simulink model "SP_nonlinear_LQR"  (R2016b)
settings: Solver=ode4  StartTime=0.0  StopTime=100  FixedStep=0.001  RelTol=1e-3
values from neighbouring files (symbols this model uses):
  K = lqr(P_sp,Q,R)    [SP_LQG_controller_design.m]
  Ke_sp = K_bar(:,1)    [SP_LQG_controller_design.m]    (also in controller_parameter.mat = -14.1421356237)
  Kx_sp = K_bar(:,2:end)    [SP_LQG_controller_design.m]    (also in controller_parameter.mat = [-9.4028503548 -29.2130812278])
undefined symbols (not defined in the file or in its folder): An, Aqw, Asp1, Bn, Bqw, Bsp1, Cn, Cqw, Csp1, Kn, lin_sys, Nu, Nu_inv, Nx, Ny, op
libraries: aerolibatmos2 x10, aerolib3dof2 x1, aerolib6dof2 x1, aerolibasang x1
(part 2 of 7)

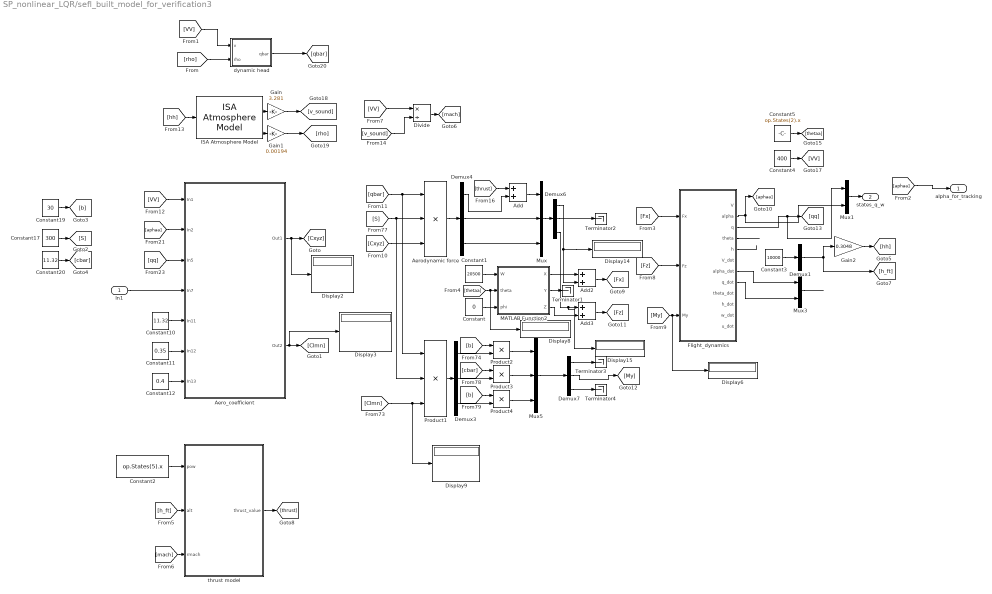
== system SP_nonlinear_LQR/sefl_built_model_for_verification3 ==
  In1 : Inport
  Add : Sum
  Add2 : Sum
  Add3 : Sum
  Aero_coefficient : Subsystem
      mask Display:
      | port_label('input', 1, 'vt')
      | port_label('input', 2, 'alpha')
      | 
      | port_label('input', 3, 'q')
      | 
      | port_label('input', 4, 'el')
      | 
      | 
      | 
      | port_label('input', 5, 'cbar')
      | port_label('input', 6, 'xcgr')
      | port_label('input', 7, 'xcg')
      | port_label('output', 1, 'Cxz')
      | port_label('output', 2, 'Cm')
  "Aerodynamic force " : Product  Inputs=3
  Constant : Constant  Value=0
  Constant1 : Constant  Value=20500
  Constant10 : Constant  Value=11.32
  Constant11 : Constant  Value=0.35
  Constant12 : Constant  Value=0.4
  Constant17 : Constant  Value=300
  Constant19 : Constant  Value=30
  Constant2 : Constant  Value=op.States(5).x
  Constant20 : Constant  Value=11.32
  Constant3 : Constant  Value=10000
  Constant4 : Constant  Value=400
  Constant5 : Constant  Value=op.States(2).x
  Demux1 : Demux  Outputs=1
  Demux{3..4,6..7} (4 alike) : Demux  Outputs=3
  Display{2..3,6,8..9,14..15} (7 alike) : Display
  Divide : Product  Inputs=*/
  Flight_dynamics : Subsystem
  Gain : Gain  Gain=3.281
  Gain1 : Gain  Gain=0.00194
  Gain2 : Gain  Gain=0.3048
  ISA Atmosphere Model : aerolibatmos2/ISA Atmosphere Model  custom=off  g=9.80665  gamma=1.4  R=287.0531  L=0.0065  h_trop=11000  h_strat=20000  rho0=1.225  P0=101325  T0=288.15  h0=0
  MATLAB Function2 : MATLAB Function  TreatAsAtomicUnit=on
  Mux : Mux  Inputs=3
  Mux1 : Mux  Inputs=2
  Mux3 : Mux  Inputs=2
  Mux5 : Mux  Inputs=3
  Product1 : Product  Inputs=3
  Product2 : Product
  Product3 : Product
  Product4 : Product
  Terminator{1..4} (4 alike) : Terminator
  dynamic head : MATLAB Function  TreatAsAtomicUnit=on
  thrust model : MATLAB Function  TreatAsAtomicUnit=on
  alpha_for_tracking : Outport
  states_q_w : Outport  Port=2
  wires:
  [aphaa] -> alpha_for_tracking/1
  Constant5/1 -> [thetaa]
  Constant4/1 -> [VV]
  Constant3/1 -> Demux1/1
  Constant2/1 -> thrust model/1(pow)
  Flight_dynamics/8(q_dot) -> Mux3/2
  Flight_dynamics/7(alpha_dot) -> Mux3/1
  [qq] -> Aero_coefficient/3(In5)
  [aphaa] -> Aero_coefficient/2(In2)
  [VV] -> Aero_coefficient/1(In1)
  Flight_dynamics/5(h) -> ?
  ISA Atmosphere Model/4 -> Gain1/1
  ISA Atmosphere Model/2 -> Gain/1
  [qbar] -> Product1/1, "Aerodynamic force "/1
  In1/1 -> Aero_coefficient/4(In7)
  Product4/1 -> Mux5/3
  Constant10/1 -> Aero_coefficient/5(In11)
  Constant11/1 -> Aero_coefficient/6(In12)
  Mux5/1 -> Demux7/1
  Constant17/1 -> [S]
  Gain1/1 -> [rho]
  Product3/1 -> Mux5/2
  Product2/1 -> Mux5/1
  [VV] -> Divide/1
  [VV] -> dynamic head/1(v)
  Aero_coefficient/1(Out1) -> Display2/1, [Cxyz]
  [rho] -> dynamic head/2(rho)
  Aero_coefficient/2(Out2) -> [Clmn], Display3/1
  Constant20/1 -> [cbar]
  Constant19/1 -> [b]
  Demux1/1 -> Gain2/1, [h_ft]
  [hh] -> ISA Atmosphere Model/1
  Demux4/3 -> Mux/3
  Gain/1 -> [v_sound]
  Divide/1 -> [mach]
  Add/1 -> Mux/1
  Demux4/2 -> Mux/2
  [v_sound] -> Divide/2
  Demux4/1 -> Add/2
  Mux/1 -> Demux6/1
  Constant12/1 -> Aero_coefficient/7(In13)
  Gain2/1 -> [hh]
  dynamic head/1(qbar) -> [qbar]
  thrust model/1(thrust_value) -> [thrust]
  [h_ft] -> thrust model/2(alt)
  [mach] -> thrust model/3(rmach)
  [thrust] -> Add/1
  Demux3/3 -> Product4/2
  [b] -> Product4/1
  "Aerodynamic force "/1 -> Demux4/1
  [Cxyz] -> "Aerodynamic force "/3
  [S] -> "Aerodynamic force "/2, Product1/2
  [Clmn] -> Display9/1, Product1/3
  [b] -> Product2/1
  Product1/1 -> Demux3/1
  Demux3/1 -> Product2/2
  Demux3/2 -> Product3/2
  [cbar] -> Product3/1
  Demux6/3 -> Display15/1, Add3/1
  Demux6/2 -> Terminator2/1
  Demux7/1 -> Terminator3/1
  Demux7/3 -> Terminator4/1
  Constant1/1 -> MATLAB Function2/1(W)
  [thetaa] -> Display8/1, MATLAB Function2/2(theta)
  Constant/1 -> MATLAB Function2/3(phi)
  MATLAB Function2/1(X) -> Add2/1
  Demux6/1 -> Display14/1, Add2/2
  MATLAB Function2/3(Z) -> Add3/2
  MATLAB Function2/2(Y) -> Terminator1/1
  Add2/1 -> [Fx]
  Add3/1 -> [Fz]
  Demux7/2 -> [My]
  [Fx] -> Flight_dynamics/1(Fx)
  [Fz] -> Flight_dynamics/2(Fz)
  [My] -> Flight_dynamics/3(My), Display6/1
  Mux3/1 -> ?
  Flight_dynamics/2(alpha) -> Mux1/2, [aphaa]
  Flight_dynamics/3(q) -> Mux1/1, [qq]
  Flight_dynamics/4(theta) -> ?
  Mux1/1 -> states_q_w/1

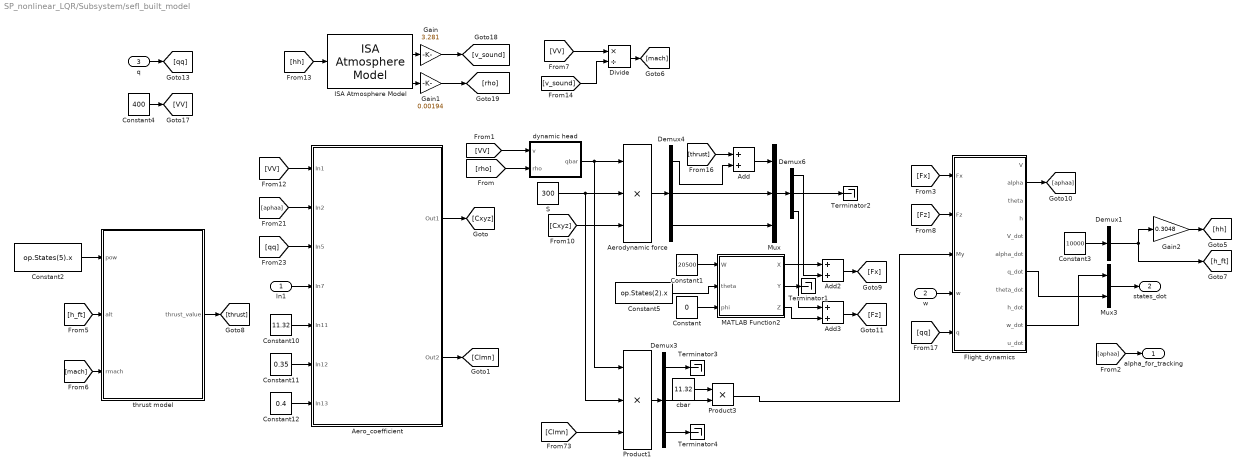
== system SP_nonlinear_LQR/Subsystem/sefl_built_model ==
  In1 : Inport
  w : Inport  Port=2
  q : Inport  Port=3
  Add : Sum
  Add2 : Sum
  Add3 : Sum
  Aero_coefficient : Subsystem
      mask Display:
      | port_label('input', 1, 'vt')
      | port_label('input', 2, 'alpha')
      | 
      | port_label('input', 3, 'q')
      | 
      | port_label('input', 4, 'el')
      | 
      | 
      | 
      | port_label('input', 5, 'cbar')
      | port_label('input', 6, 'xcgr')
      | port_label('input', 7, 'xcg')
      | port_label('output', 1, 'Cxz')
      | port_label('output', 2, 'Cm')
  "Aerodynamic force " : Product  Inputs=3
  Constant : Constant  Value=0
  Constant1 : Constant  Value=20500
  Constant10 : Constant  Value=11.32
  Constant11 : Constant  Value=0.35
  Constant12 : Constant  Value=0.4
  Constant2 : Constant  Value=op.States(5).x
  Constant3 : Constant  Value=10000
  Constant4 : Constant  Value=400
  Constant5 : Constant  Value=op.States(2).x
  Demux1 : Demux  Outputs=1
  Demux3 : Demux  Outputs=3
  Demux4 : Demux  Outputs=3
  Demux6 : Demux  Outputs=3
  Divide : Product  Inputs=*/
  Flight_dynamics : Subsystem
  Gain : Gain  Gain=3.281
  Gain1 : Gain  Gain=0.00194
  Gain2 : Gain  Gain=0.3048
  ISA Atmosphere Model : aerolibatmos2/ISA Atmosphere Model  custom=off  g=9.80665  gamma=1.4  R=287.0531  L=0.0065  h_trop=11000  h_strat=20000  rho0=1.225  P0=101325  T0=288.15  h0=0
  MATLAB Function2 : MATLAB Function  TreatAsAtomicUnit=on
  Mux : Mux  Inputs=3
  Mux3 : Mux  Inputs=2
  Product1 : Product  Inputs=3
  Product3 : Product
  S : Constant  Value=300
  Terminator{1..4} (4 alike) : Terminator
  cbar : Constant  Value=11.32
  dynamic head : MATLAB Function  TreatAsAtomicUnit=on
  thrust model : MATLAB Function  TreatAsAtomicUnit=on
  alpha_for_tracking : Outport
  states_dot : Outport  Port=2
  wires:
  Flight_dynamics/2(alpha) -> [aphaa]
  Mux3/1 -> states_dot/1
  Product3/1 -> Flight_dynamics/3(My)
  [Fz] -> Flight_dynamics/2(Fz)
  [Fx] -> Flight_dynamics/1(Fx)
  Add3/1 -> [Fz]
  Add2/1 -> [Fx]
  MATLAB Function2/2(Y) -> Terminator1/1
  MATLAB Function2/3(Z) -> Add3/2
  Demux6/1 -> Add2/2
  MATLAB Function2/1(X) -> Add2/1
  Constant/1 -> MATLAB Function2/3(phi)
  Constant5/1 -> MATLAB Function2/2(theta)
  Constant1/1 -> MATLAB Function2/1(W)
  Demux6/2 -> Terminator2/1
  Demux6/3 -> Add3/1
  cbar/1 -> Product3/1
  Demux3/2 -> Product3/2
  Product1/1 -> Demux3/1
  [Clmn] -> Product1/3
  S/1 -> Product1/2, "Aerodynamic force "/2
  [Cxyz] -> "Aerodynamic force "/3
  "Aerodynamic force "/1 -> Demux4/1
  [thrust] -> Add/1
  [mach] -> thrust model/3(rmach)
  [h_ft] -> thrust model/2(alt)
  thrust model/1(thrust_value) -> [thrust]
  Gain2/1 -> [hh]
  Constant12/1 -> Aero_coefficient/7(In13)
  Mux/1 -> Demux6/1
  Demux4/1 -> Add/2
  [v_sound] -> Divide/2
  Demux4/2 -> Mux/2
  Add/1 -> Mux/1
  Divide/1 -> [mach]
  Gain/1 -> [v_sound]
  Demux4/3 -> Mux/3
  [hh] -> ISA Atmosphere Model/1
  Demux1/1 -> [h_ft], Gain2/1
  Aero_coefficient/2(Out2) -> [Clmn]
  [rho] -> dynamic head/2(rho)
  Aero_coefficient/1(Out1) -> [Cxyz]
  [VV] -> dynamic head/1(v)
  [VV] -> Divide/1
  Gain1/1 -> [rho]
  Constant11/1 -> Aero_coefficient/6(In12)
  Constant10/1 -> Aero_coefficient/5(In11)
  In1/1 -> Aero_coefficient/4(In7)
  dynamic head/1(qbar) -> "Aerodynamic force "/1, Product1/1
  ISA Atmosphere Model/2 -> Gain/1
  ISA Atmosphere Model/4 -> Gain1/1
  [VV] -> Aero_coefficient/1(In1)
  [aphaa] -> Aero_coefficient/2(In2)
  [qq] -> Aero_coefficient/3(In5)
  q/1 -> [qq]
  Flight_dynamics/10(w_dot) -> Mux3/1
  Flight_dynamics/7(q_dot) -> Mux3/2
  Constant2/1 -> thrust model/1(pow)
  Constant3/1 -> Demux1/1
  Constant4/1 -> [VV]
  [aphaa] -> alpha_for_tracking/1
  w/1 -> Flight_dynamics/4(w)
  [qq] -> Flight_dynamics/5(q)
  Demux3/1 -> Terminator3/1
  Demux3/3 -> Terminator4/1

== system SP_nonlinear_LQR/Subsystem1/Aero_coefficient ==
  In1 : Inport
  In2 : Inport  Port=2
  In5 : Inport  Port=3
  In7 : Inport  Port=4
  In11 : Inport  Port=5
  In12 : Inport  Port=6
  In13 : Inport  Port=7
  Aerodynamic coefficient : MATLAB Function  TreatAsAtomicUnit=on
  Constant : Constant
  Constant1 : Constant
  Constant2 : Constant
  Mux1 : Mux  Inputs=3
  Mux2 : Mux  Inputs=3
  Out1 : Outport
  Out2 : Outport  Port=2
  wires:
  In5/1 -> Aerodynamic coefficient/3(q)
  In1/1 -> Aerodynamic coefficient/1(vt)
  In2/1 -> Aerodynamic coefficient/2(alpha)
  In7/1 -> Aerodynamic coefficient/4(el)
  Aerodynamic coefficient/3(cmt) -> Mux2/2
  In11/1 -> Aerodynamic coefficient/5(cbar)
  In12/1 -> Aerodynamic coefficient/6(xcgr)
  Aerodynamic coefficient/2(czt) -> Mux1/3
  In13/1 -> Aerodynamic coefficient/7(xcg)
  Aerodynamic coefficient/1(cxt) -> Mux1/1
  Mux1/1 -> Out1/1
  Mux2/1 -> Out2/1
  Constant/1 -> Mux1/2
  Constant1/1 -> Mux2/1
  Constant2/1 -> Mux2/3

== system SP_nonlinear_LQR/dynamic_for_linsys1/Aero_coefficient ==
  In1 : Inport
  In2 : Inport  Port=2
  In5 : Inport  Port=3
  In7 : Inport  Port=4
  In11 : Inport  Port=5
  In12 : Inport  Port=6
  In13 : Inport  Port=7
  Aerodynamic coefficient : MATLAB Function  TreatAsAtomicUnit=on
  Constant : Constant
  Constant1 : Constant
  Constant2 : Constant
  Mux1 : Mux  Inputs=3
  Mux2 : Mux  Inputs=3
  Out1 : Outport
  Out2 : Outport  Port=2
  wires:
  In5/1 -> Aerodynamic coefficient/3(q)
  In1/1 -> Aerodynamic coefficient/1(vt)
  In2/1 -> Aerodynamic coefficient/2(alpha)
  In7/1 -> Aerodynamic coefficient/4(el)
  Aerodynamic coefficient/3(cmt) -> Mux2/2
  In11/1 -> Aerodynamic coefficient/5(cbar)
  In12/1 -> Aerodynamic coefficient/6(xcgr)
  Aerodynamic coefficient/2(czt) -> Mux1/3
  In13/1 -> Aerodynamic coefficient/7(xcg)
  Aerodynamic coefficient/1(cxt) -> Mux1/1
  Mux1/1 -> Out1/1
  Mux2/1 -> Out2/1
  Constant/1 -> Mux1/2
  Constant1/1 -> Mux2/1
  Constant2/1 -> Mux2/3

== system SP_nonlinear_LQR/dynamic_for_linsys1/Flight_dynamics ==
  Fx : Inport
  Fz : Inport  Port=2
  My : Inport  Port=3
  Display : Display
  From8 : From  Commented=on  GotoTag=h
  From9 : From  Commented=on  GotoTag=w
  Gain : Gain  Gain=1.57e-3
  Gain1 : Gain  Gain=1.57e-3
  Gain2 : Gain  Gain=1/55814
  Goto15 : Goto  Commented=on  GotoTag=h
  Integrator : Integrator  InitialCondition=op.States(3).x(1)
  Integrator1 : Integrator  InitialCondition=op.States(3).x(2)
  Integrator2 : Integrator
  Integrator3 : Integrator  InitialCondition=op.States(2).x
  Integrator4 : Integrator  Commented=on  InitialCondition=10000
  MATLAB Function : MATLAB Function  TreatAsAtomicUnit=on
  Product : Product
  Product1 : Product
  Sum : Sum  Inputs=|-+
  Sum1 : Sum  Inputs=|++
  V : Outport
  alpha : Outport  Port=2
  q : Outport  Port=3
  theta : Outport  Port=4
  V_dot : Outport  Port=5
  alpha_dot : Outport  Port=6
  q_dot : Outport  Port=7
  theta_dot : Outport  Port=8
  wires:
  Fx/1 -> Gain/1
  Fz/1 -> Gain1/1
  Gain/1 -> [Fx_m]
  Gain1/1 -> [Fz_m]
  My/1 -> Gain2/1
  Gain2/1 -> [My_Iy]
  Product/1 -> Sum/1
  [Fx_m] -> Sum/2
  Sum/1 -> [u_dot], Integrator/1  "u_dot"
  Integrator/1 -> [u], Product1/1  "u"
  Product1/1 -> Sum1/1
  [Fz_m] -> Sum1/2
  Sum1/1 -> [w_dot], Integrator1/1  "w_dot"
  Integrator1/1 -> Integrator4/1, [w]  "w"
  [w] -> Product/2
  [My_Iy] -> [q], Integrator2/1  "q_dot"
  Integrator2/1 -> Product1/2, [q_dot], [theta_dot], Integrator3/1, Product/1  "q"
  Integrator3/1 -> [theta]  "theta"
  [w] -> MATLAB Function/1(w)
  MATLAB Function/2(alpha) -> [alpha]
  [u_dot] -> MATLAB Function/4(u_dot)
  [w_dot] -> MATLAB Function/3(w_dot)
  MATLAB Function/3(alpha_dot) -> [alpha_dot]
  [V] -> Display/1, V/1
  [alpha] -> alpha/1
  [q] -> q/1
  [theta] -> theta/1
  [V_dot] -> V_dot/1
  [alpha_dot] -> alpha_dot/1
  [q_dot] -> q_dot/1
  [theta_dot] -> theta_dot/1
  MATLAB Function/1(V) -> [V]
  MATLAB Function/4(V_dot) -> [V_dot]
  Integrator4/1 -> Goto15/1
  From9/1 -> ?
  [u] -> MATLAB Function/2(u)

== system SP_nonlinear_LQR/q_w_as states/Aero_coefficient ==
  In1 : Inport
  In2 : Inport  Port=2
  In5 : Inport  Port=3
  In7 : Inport  Port=4
  In11 : Inport  Port=5
  In12 : Inport  Port=6
  In13 : Inport  Port=7
  Aerodynamic coefficient : MATLAB Function  TreatAsAtomicUnit=on
  Constant : Constant
  Constant1 : Constant
  Constant2 : Constant
  Mux1 : Mux  Inputs=3
  Mux2 : Mux  Inputs=3
  Out1 : Outport
  Out2 : Outport  Port=2
  wires:
  In5/1 -> Aerodynamic coefficient/3(q)
  In1/1 -> Aerodynamic coefficient/1(vt)
  In2/1 -> Aerodynamic coefficient/2(alpha)
  In7/1 -> Aerodynamic coefficient/4(el)
  Aerodynamic coefficient/3(cmt) -> Mux2/2
  In11/1 -> Aerodynamic coefficient/5(cbar)
  In12/1 -> Aerodynamic coefficient/6(xcgr)
  Aerodynamic coefficient/2(czt) -> Mux1/3
  In13/1 -> Aerodynamic coefficient/7(xcg)
  Aerodynamic coefficient/1(cxt) -> Mux1/1
  Mux1/1 -> Out1/1
  Mux2/1 -> Out2/1
  Constant/1 -> Mux1/2
  Constant1/1 -> Mux2/1
  Constant2/1 -> Mux2/3

== system SP_nonlinear_LQR/q_w_as states/Flight_dynamics ==
  Fx : Inport
  Fz : Inport  Port=2
  My : Inport  Port=3
  Constant : Constant  Value=op.States(3).x(1)
  Constant1 : Constant  Value=0
  Display : Display
  Gain : Gain  Gain=1/637.1604
  Gain1 : Gain  Gain=1/637.1604
  Gain2 : Gain  Gain=1/55814
  Goto15 : Goto  Commented=on  GotoTag=h
  Goto4 : Goto  Commented=on  GotoTag=theta
  Goto5 : Goto  Commented=on  GotoTag=theta_dot
  Integrator1 : Integrator  InitialCondition=op.States(3).x(2)
  Integrator2 : Integrator
  Integrator3 : Integrator  Commented=on  InitialCondition=op.States(2).x
  Integrator4 : Integrator  Commented=on  InitialCondition=10000
  MATLAB Function : MATLAB Function  TreatAsAtomicUnit=on
  Product1 : Product
  Sum1 : Sum  Inputs=|++
  V : Outport
  alpha : Outport  Port=2
  q : Outport  Port=3
  theta : Outport  Port=4
  h : Outport  Port=5
  V_dot : Outport  Port=6
  alpha_dot : Outport  Port=7
  q_dot : Outport  Port=8
  theta_dot : Outport  Port=9
  h_dot : Outport  Port=10
  w_dot : Outport  Port=11
  u_dot : Outport  Port=12
  wires:
  [u] -> Product1/1
  Constant1/1 -> MATLAB Function/4(u_dot)
  Constant/1 -> [u]
  Fx/1 -> Gain/1
  Fz/1 -> Gain1/1
  Gain/1 -> [Fx_m]
  Gain1/1 -> [Fz_m]
  My/1 -> Gain2/1
  Gain2/1 -> [My_Iy]
  Product1/1 -> Sum1/1
  [Fz_m] -> Sum1/2
  Sum1/1 -> Integrator1/1, [w_dot]  "w_dot"
  Integrator1/1 -> Integrator4/1, [w]  "w"
  [My_Iy] -> [q_dot], Integrator2/1  "q_dot"
  Integrator2/1 -> Product1/2, [q], Goto5/1, Integrator3/1  "q"
  Integrator3/1 -> Goto4/1  "theta"
  [w] -> MATLAB Function/1(w)
  MATLAB Function/2(alpha) -> [alpha]
  [w_dot] -> MATLAB Function/3(w_dot)
  MATLAB Function/3(alpha_dot) -> [alpha_dot]
  [V] -> Display/1, V/1
  [alpha] -> alpha/1
  [q] -> q/1
  [theta] -> theta/1
  [V_dot] -> V_dot/1
  [alpha_dot] -> alpha_dot/1
  [q_dot] -> q_dot/1
  [theta_dot] -> theta_dot/1
  MATLAB Function/1(V) -> [V]
  MATLAB Function/4(V_dot) -> [V_dot]
  Integrator4/1 -> Goto15/1
  [h] -> h/1
  [w] -> h_dot/1
  [u] -> MATLAB Function/2(u)
  [w_dot] -> w_dot/1
  [u_dot] -> u_dot/1

== system SP_nonlinear_LQR/q_w_as states1/Aero_coefficient ==
  In1 : Inport
  In2 : Inport  Port=2
  In5 : Inport  Port=3
  In7 : Inport  Port=4
  In11 : Inport  Port=5
  In12 : Inport  Port=6
  In13 : Inport  Port=7
  Aerodynamic coefficient : MATLAB Function  TreatAsAtomicUnit=on
  Constant : Constant
  Constant1 : Constant
  Constant2 : Constant
  Mux1 : Mux  Inputs=3
  Mux2 : Mux  Inputs=3
  Out1 : Outport
  Out2 : Outport  Port=2
  wires:
  In5/1 -> Aerodynamic coefficient/3(q)
  In1/1 -> Aerodynamic coefficient/1(vt)
  In2/1 -> Aerodynamic coefficient/2(alpha)
  In7/1 -> Aerodynamic coefficient/4(el)
  Aerodynamic coefficient/3(cmt) -> Mux2/2
  In11/1 -> Aerodynamic coefficient/5(cbar)
  In12/1 -> Aerodynamic coefficient/6(xcgr)
  Aerodynamic coefficient/2(czt) -> Mux1/3
  In13/1 -> Aerodynamic coefficient/7(xcg)
  Aerodynamic coefficient/1(cxt) -> Mux1/1
  Mux1/1 -> Out1/1
  Mux2/1 -> Out2/1
  Constant/1 -> Mux1/2
  Constant1/1 -> Mux2/1
  Constant2/1 -> Mux2/3

== system SP_nonlinear_LQR/q_w_as states1/Flight_dynamics ==
  Fx : Inport
  Fz : Inport  Port=2
  My : Inport  Port=3
  Constant : Constant  Value=op.States(3).x(1)
  Constant1 : Constant  Value=0
  Display : Display
  Gain : Gain  Gain=1/637.1604
  Gain1 : Gain  Gain=1/637.1604
  Gain2 : Gain  Gain=1/55814
  Goto15 : Goto  Commented=on  GotoTag=h
  Goto4 : Goto  Commented=on  GotoTag=theta
  Goto5 : Goto  Commented=on  GotoTag=theta_dot
  Integrator1 : Integrator  InitialCondition=op.States(3).x(2)
  Integrator2 : Integrator
  Integrator3 : Integrator  Commented=on  InitialCondition=op.States(2).x
  Integrator4 : Integrator  Commented=on  InitialCondition=10000
  MATLAB Function : MATLAB Function  TreatAsAtomicUnit=on
  Product1 : Product
  Sum1 : Sum  Inputs=|++
  V : Outport
  alpha : Outport  Port=2
  q : Outport  Port=3
  theta : Outport  Port=4
  h : Outport  Port=5
  V_dot : Outport  Port=6
  alpha_dot : Outport  Port=7
  q_dot : Outport  Port=8
  theta_dot : Outport  Port=9
  h_dot : Outport  Port=10
  w_dot : Outport  Port=11
  u_dot : Outport  Port=12
  wires:
  [u] -> Product1/1
  Constant1/1 -> MATLAB Function/4(u_dot)
  Constant/1 -> [u]
  Fx/1 -> Gain/1
  Fz/1 -> Gain1/1
  Gain/1 -> [Fx_m]
  Gain1/1 -> [Fz_m]
  My/1 -> Gain2/1
  Gain2/1 -> [My_Iy]
  Product1/1 -> Sum1/1
  [Fz_m] -> Sum1/2
  Sum1/1 -> Integrator1/1, [w_dot]  "w_dot"
  Integrator1/1 -> Integrator4/1, [w]  "w"
  [My_Iy] -> [q_dot], Integrator2/1  "q_dot"
  Integrator2/1 -> Product1/2, [q], Goto5/1, Integrator3/1  "q"
  Integrator3/1 -> Goto4/1  "theta"
  [w] -> MATLAB Function/1(w)
  MATLAB Function/2(alpha) -> [alpha]
  [w_dot] -> MATLAB Function/3(w_dot)
  MATLAB Function/3(alpha_dot) -> [alpha_dot]
  [V] -> Display/1, V/1
  [alpha] -> alpha/1
  [q] -> q/1
  [theta] -> theta/1
  [V_dot] -> V_dot/1
  [alpha_dot] -> alpha_dot/1
  [q_dot] -> q_dot/1
  [theta_dot] -> theta_dot/1
  MATLAB Function/1(V) -> [V]
  MATLAB Function/4(V_dot) -> [V_dot]
  Integrator4/1 -> Goto15/1
  [h] -> h/1
  [w] -> h_dot/1
  [u] -> MATLAB Function/2(u)
  [w_dot] -> w_dot/1
  [u_dot] -> u_dot/1

== system SP_nonlinear_LQR/q_w_as states2/Aero_coefficient ==
  In1 : Inport
  In2 : Inport  Port=2
  In5 : Inport  Port=3
  In7 : Inport  Port=4
  In11 : Inport  Port=5
  In12 : Inport  Port=6
  In13 : Inport  Port=7
  Aerodynamic coefficient : MATLAB Function  TreatAsAtomicUnit=on
  Constant : Constant
  Constant1 : Constant
  Constant2 : Constant
  Mux1 : Mux  Inputs=3
  Mux2 : Mux  Inputs=3
  Out1 : Outport
  Out2 : Outport  Port=2
  wires:
  In5/1 -> Aerodynamic coefficient/3(q)
  In1/1 -> Aerodynamic coefficient/1(vt)
  In2/1 -> Aerodynamic coefficient/2(alpha)
  In7/1 -> Aerodynamic coefficient/4(el)
  Aerodynamic coefficient/3(cmt) -> Mux2/2
  In11/1 -> Aerodynamic coefficient/5(cbar)
  In12/1 -> Aerodynamic coefficient/6(xcgr)
  Aerodynamic coefficient/2(czt) -> Mux1/3
  In13/1 -> Aerodynamic coefficient/7(xcg)
  Aerodynamic coefficient/1(cxt) -> Mux1/1
  Mux1/1 -> Out1/1
  Mux2/1 -> Out2/1
  Constant/1 -> Mux1/2
  Constant1/1 -> Mux2/1
  Constant2/1 -> Mux2/3

== system SP_nonlinear_LQR/q_w_as states2/Flight_dynamics ==
  Fx : Inport
  Fz : Inport  Port=2
  My : Inport  Port=3
  Constant : Constant  Value=op.States(3).x(1)
  Constant1 : Constant  Value=0
  Display : Display
  Gain : Gain  Gain=1/637.1604
  Gain1 : Gain  Gain=1/637.1604
  Gain2 : Gain  Gain=1/55814
  Goto15 : Goto  Commented=on  GotoTag=h
  Goto4 : Goto  Commented=on  GotoTag=theta
  Goto5 : Goto  Commented=on  GotoTag=theta_dot
  Integrator1 : Integrator  InitialCondition=op.States(3).x(2)
  Integrator2 : Integrator
  Integrator3 : Integrator  Commented=on  InitialCondition=op.States(2).x
  Integrator4 : Integrator  Commented=on  InitialCondition=10000
  MATLAB Function : MATLAB Function  TreatAsAtomicUnit=on
  Product1 : Product
  Sum1 : Sum  Inputs=|++
  V : Outport
  alpha : Outport  Port=2
  q : Outport  Port=3
  theta : Outport  Port=4
  h : Outport  Port=5
  V_dot : Outport  Port=6
  alpha_dot : Outport  Port=7
  q_dot : Outport  Port=8
  theta_dot : Outport  Port=9
  h_dot : Outport  Port=10
  w_dot : Outport  Port=11
  u_dot : Outport  Port=12
  wires:
  [u] -> Product1/1
  Constant1/1 -> MATLAB Function/4(u_dot)
  Constant/1 -> [u]
  Fx/1 -> Gain/1
  Fz/1 -> Gain1/1
  Gain/1 -> [Fx_m]
  Gain1/1 -> [Fz_m]
  My/1 -> Gain2/1
  Gain2/1 -> [My_Iy]
  Product1/1 -> Sum1/1
  [Fz_m] -> Sum1/2
  Sum1/1 -> Integrator1/1, [w_dot]  "w_dot"
  Integrator1/1 -> Integrator4/1, [w]  "w"
  [My_Iy] -> [q_dot], Integrator2/1  "q_dot"
  Integrator2/1 -> Product1/2, [q], Goto5/1, Integrator3/1  "q"
  Integrator3/1 -> Goto4/1  "theta"
  [w] -> MATLAB Function/1(w)
  MATLAB Function/2(alpha) -> [alpha]
  [w_dot] -> MATLAB Function/3(w_dot)
  MATLAB Function/3(alpha_dot) -> [alpha_dot]
  [V] -> Display/1, V/1
  [alpha] -> alpha/1
  [q] -> q/1
  [theta] -> theta/1
  [V_dot] -> V_dot/1
  [alpha_dot] -> alpha_dot/1
  [q_dot] -> q_dot/1
  [theta_dot] -> theta_dot/1
  MATLAB Function/1(V) -> [V]
  MATLAB Function/4(V_dot) -> [V_dot]
  Integrator4/1 -> Goto15/1
  [h] -> h/1
  [w] -> h_dot/1
  [u] -> MATLAB Function/2(u)
  [w_dot] -> w_dot/1
  [u_dot] -> u_dot/1

== system SP_nonlinear_LQR/q_w_as states3/Aero_coefficient ==
  In1 : Inport
  In2 : Inport  Port=2
  In5 : Inport  Port=3
  In7 : Inport  Port=4
  In11 : Inport  Port=5
  In12 : Inport  Port=6
  In13 : Inport  Port=7
  Aerodynamic coefficient : MATLAB Function  TreatAsAtomicUnit=on
  Constant : Constant
  Constant1 : Constant
  Constant2 : Constant
  Mux1 : Mux  Inputs=3
  Mux2 : Mux  Inputs=3
  Out1 : Outport
  Out2 : Outport  Port=2
  wires:
  In5/1 -> Aerodynamic coefficient/3(q)
  In1/1 -> Aerodynamic coefficient/1(vt)
  In2/1 -> Aerodynamic coefficient/2(alpha)
  In7/1 -> Aerodynamic coefficient/4(el)
  Aerodynamic coefficient/3(cmt) -> Mux2/2
  In11/1 -> Aerodynamic coefficient/5(cbar)
  In12/1 -> Aerodynamic coefficient/6(xcgr)
  Aerodynamic coefficient/2(czt) -> Mux1/3
  In13/1 -> Aerodynamic coefficient/7(xcg)
  Aerodynamic coefficient/1(cxt) -> Mux1/1
  Mux1/1 -> Out1/1
  Mux2/1 -> Out2/1
  Constant/1 -> Mux1/2
  Constant1/1 -> Mux2/1
  Constant2/1 -> Mux2/3

== system SP_nonlinear_LQR/q_w_as states3/Flight_dynamics ==
  Fx : Inport
  Fz : Inport  Port=2
  My : Inport  Port=3
  Constant : Constant  Value=op.States(3).x(1)
  Constant1 : Constant  Value=0
  Display : Display
  Gain : Gain  Gain=1/637.1604
  Gain1 : Gain  Gain=1/637.1604
  Gain2 : Gain  Gain=1/55814
  Goto15 : Goto  Commented=on  GotoTag=h
  Goto4 : Goto  Commented=on  GotoTag=theta
  Goto5 : Goto  Commented=on  GotoTag=theta_dot
  Integrator1 : Integrator  InitialCondition=op.States(3).x(2)
  Integrator2 : Integrator
  Integrator3 : Integrator  Commented=on  InitialCondition=op.States(2).x
  Integrator4 : Integrator  Commented=on  InitialCondition=10000
  MATLAB Function : MATLAB Function  TreatAsAtomicUnit=on
  Product1 : Product
  Sum1 : Sum  Inputs=|++
  V : Outport
  alpha : Outport  Port=2
  q : Outport  Port=3
  theta : Outport  Port=4
  h : Outport  Port=5
  V_dot : Outport  Port=6
  alpha_dot : Outport  Port=7
  q_dot : Outport  Port=8
  theta_dot : Outport  Port=9
  h_dot : Outport  Port=10
  w_dot : Outport  Port=11
  u_dot : Outport  Port=12
  wires:
  [u] -> Product1/1
  Constant1/1 -> MATLAB Function/4(u_dot)
  Constant/1 -> [u]
  Fx/1 -> Gain/1
  Fz/1 -> Gain1/1
  Gain/1 -> [Fx_m]
  Gain1/1 -> [Fz_m]
  My/1 -> Gain2/1
  Gain2/1 -> [My_Iy]
  Product1/1 -> Sum1/1
  [Fz_m] -> Sum1/2
  Sum1/1 -> Integrator1/1, [w_dot]  "w_dot"
  Integrator1/1 -> Integrator4/1, [w]  "w"
  [My_Iy] -> [q_dot], Integrator2/1  "q_dot"
  Integrator2/1 -> Product1/2, [q], Goto5/1, Integrator3/1  "q"
  Integrator3/1 -> Goto4/1  "theta"
  [w] -> MATLAB Function/1(w)
  MATLAB Function/2(alpha) -> [alpha]
  [w_dot] -> MATLAB Function/3(w_dot)
  MATLAB Function/3(alpha_dot) -> [alpha_dot]
  [V] -> Display/1, V/1
  [alpha] -> alpha/1
  [q] -> q/1
  [theta] -> theta/1
  [V_dot] -> V_dot/1
  [alpha_dot] -> alpha_dot/1
  [q_dot] -> q_dot/1
  [theta_dot] -> theta_dot/1
  MATLAB Function/1(V) -> [V]
  MATLAB Function/4(V_dot) -> [V_dot]
  Integrator4/1 -> Goto15/1
  [h] -> h/1
  [w] -> h_dot/1
  [u] -> MATLAB Function/2(u)
  [w_dot] -> w_dot/1
  [u_dot] -> u_dot/1

== system SP_nonlinear_LQR/sefl_built_model_for_verification1/Aero_coefficient ==
  In1 : Inport
  In2 : Inport  Port=2
  In5 : Inport  Port=3
  In7 : Inport  Port=4
  In11 : Inport  Port=5
  In12 : Inport  Port=6
  In13 : Inport  Port=7
  Aerodynamic coefficient : MATLAB Function  TreatAsAtomicUnit=on
  Constant : Constant
  Constant1 : Constant
  Constant2 : Constant
  Mux1 : Mux  Inputs=3
  Mux2 : Mux  Inputs=3
  Out1 : Outport
  Out2 : Outport  Port=2
  wires:
  Constant2/1 -> Mux2/3
  Constant1/1 -> Mux2/1
  Constant/1 -> Mux1/2
  Mux2/1 -> Out2/1
  Mux1/1 -> Out1/1
  Aerodynamic coefficient/1(cxt) -> Mux1/1
  In13/1 -> Aerodynamic coefficient/7(xcg)
  Aerodynamic coefficient/2(czt) -> Mux1/3
  In12/1 -> Aerodynamic coefficient/6(xcgr)
  In11/1 -> Aerodynamic coefficient/5(cbar)
  Aerodynamic coefficient/3(cmt) -> Mux2/2
  In7/1 -> Aerodynamic coefficient/4(el)
  In2/1 -> Aerodynamic coefficient/2(alpha)
  In1/1 -> Aerodynamic coefficient/1(vt)
  In5/1 -> Aerodynamic coefficient/3(q)

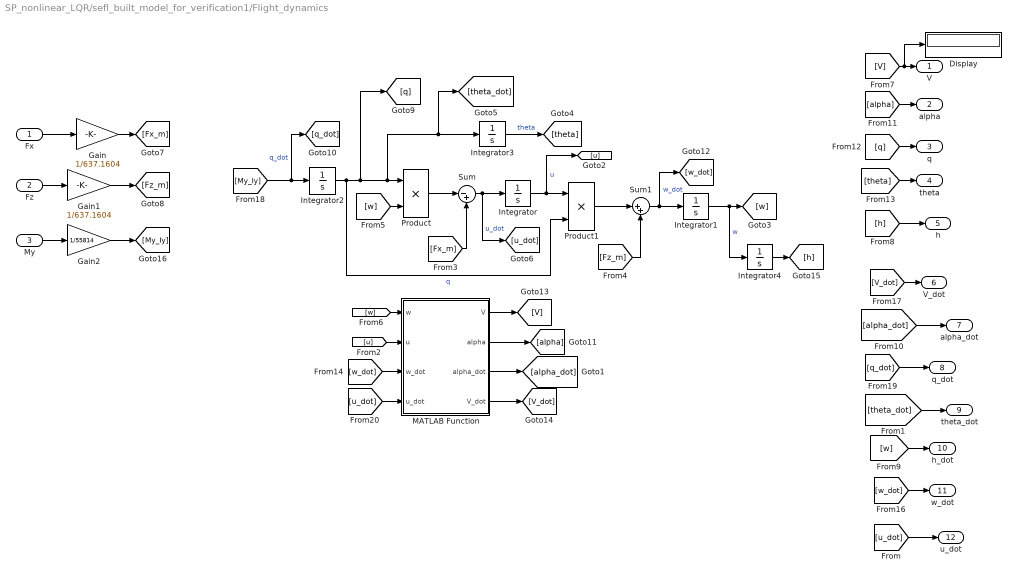
== system SP_nonlinear_LQR/sefl_built_model_for_verification1/Flight_dynamics ==
  Fx : Inport
  Fz : Inport  Port=2
  My : Inport  Port=3
  Display : Display
  Gain : Gain  Gain=1/637.1604
  Gain1 : Gain  Gain=1/637.1604
  Gain2 : Gain  Gain=1/55814
  Integrator : Integrator  InitialCondition=op.States(3).x(1)
  Integrator1 : Integrator  InitialCondition=op.States(3).x(2)
  Integrator2 : Integrator
  Integrator3 : Integrator  InitialCondition=op.States(2).x
  Integrator4 : Integrator  InitialCondition=10000
  MATLAB Function : MATLAB Function  TreatAsAtomicUnit=on
  Product : Product
  Product1 : Product
  Sum : Sum  Inputs=|-+
  Sum1 : Sum  Inputs=|++
  V : Outport
  alpha : Outport  Port=2
  q : Outport  Port=3
  theta : Outport  Port=4
  h : Outport  Port=5
  V_dot : Outport  Port=6
  alpha_dot : Outport  Port=7
  q_dot : Outport  Port=8
  theta_dot : Outport  Port=9
  h_dot : Outport  Port=10
  w_dot : Outport  Port=11
  u_dot : Outport  Port=12
  wires:
  [u_dot] -> u_dot/1
  [w_dot] -> w_dot/1
  [u] -> MATLAB Function/2(u)
  [w] -> h_dot/1
  [h] -> h/1
  Integrator4/1 -> [h]
  MATLAB Function/4(V_dot) -> [V_dot]
  MATLAB Function/1(V) -> [V]
  [theta_dot] -> theta_dot/1
  [q_dot] -> q_dot/1
  [alpha_dot] -> alpha_dot/1
  [V_dot] -> V_dot/1
  [theta] -> theta/1
  [q] -> q/1
  [alpha] -> alpha/1
  [V] -> V/1, Display/1
  MATLAB Function/3(alpha_dot) -> [alpha_dot]
  [w_dot] -> MATLAB Function/3(w_dot)
  [u_dot] -> MATLAB Function/4(u_dot)
  MATLAB Function/2(alpha) -> [alpha]
  [w] -> MATLAB Function/1(w)
  Integrator3/1 -> [theta]  "theta"
  Integrator2/1 -> Product/1, Integrator3/1, [theta_dot], [q], Product1/2  "q"
  [My_Iy] -> Integrator2/1, [q_dot]  "q_dot"
  [w] -> Product/2
  Integrator1/1 -> [w], Integrator4/1  "w"
  Sum1/1 -> Integrator1/1, [w_dot]  "w_dot"
  [Fz_m] -> Sum1/2
  Product1/1 -> Sum1/1
  Integrator/1 -> Product1/1, [u]  "u"
  Sum/1 -> Integrator/1, [u_dot]  "u_dot"
  [Fx_m] -> Sum/2
  Product/1 -> Sum/1
  Gain2/1 -> [My_Iy]
  My/1 -> Gain2/1
  Gain1/1 -> [Fz_m]
  Gain/1 -> [Fx_m]
  Fz/1 -> Gain1/1
  Fx/1 -> Gain/1

== system SP_nonlinear_LQR/sefl_built_model_for_verification2/Aero_coefficient ==
  In1 : Inport
  In2 : Inport  Port=2
  In5 : Inport  Port=3
  In7 : Inport  Port=4
  In11 : Inport  Port=5
  In12 : Inport  Port=6
  In13 : Inport  Port=7
  Aerodynamic coefficient : MATLAB Function  TreatAsAtomicUnit=on
  Constant : Constant
  Constant1 : Constant
  Constant2 : Constant
  Mux1 : Mux  Inputs=3
  Mux2 : Mux  Inputs=3
  Out1 : Outport
  Out2 : Outport  Port=2
  wires:
  In5/1 -> Aerodynamic coefficient/3(q)
  In1/1 -> Aerodynamic coefficient/1(vt)
  In2/1 -> Aerodynamic coefficient/2(alpha)
  In7/1 -> Aerodynamic coefficient/4(el)
  Aerodynamic coefficient/3(cmt) -> Mux2/2
  In11/1 -> Aerodynamic coefficient/5(cbar)
  In12/1 -> Aerodynamic coefficient/6(xcgr)
  Aerodynamic coefficient/2(czt) -> Mux1/3
  In13/1 -> Aerodynamic coefficient/7(xcg)
  Aerodynamic coefficient/1(cxt) -> Mux1/1
  Mux1/1 -> Out1/1
  Mux2/1 -> Out2/1
  Constant/1 -> Mux1/2
  Constant1/1 -> Mux2/1
  Constant2/1 -> Mux2/3

== system SP_nonlinear_LQR/sefl_built_model_for_verification2/Flight_dynamics ==
  Fx : Inport
  Fz : Inport  Port=2
  My : Inport  Port=3
  Constant : Constant  Value=op.States(3).x(1)
  Constant1 : Constant  Value=0
  Display : Display
  Gain : Gain  Gain=1/637.1604
  Gain1 : Gain  Gain=1/637.1604
  Gain2 : Gain  Gain=1/55814
  Goto15 : Goto  Commented=on  GotoTag=h
  Goto4 : Goto  Commented=on  GotoTag=theta
  Goto5 : Goto  Commented=on  GotoTag=theta_dot
  Integrator1 : Integrator  InitialCondition=op.States(3).x(2)
  Integrator2 : Integrator
  Integrator3 : Integrator  Commented=on  InitialCondition=op.States(2).x
  Integrator4 : Integrator  Commented=on  InitialCondition=10000
  MATLAB Function : MATLAB Function  TreatAsAtomicUnit=on
  Product1 : Product
  Sum1 : Sum  Inputs=|++
  V : Outport
  alpha : Outport  Port=2
  q : Outport  Port=3
  theta : Outport  Port=4
  h : Outport  Port=5
  V_dot : Outport  Port=6
  alpha_dot : Outport  Port=7
  q_dot : Outport  Port=8
  theta_dot : Outport  Port=9
  h_dot : Outport  Port=10
  w_dot : Outport  Port=11
  u_dot : Outport  Port=12
  wires:
  [u] -> Product1/1
  Constant1/1 -> MATLAB Function/4(u_dot)
  Constant/1 -> [u]
  Fx/1 -> Gain/1
  Fz/1 -> Gain1/1
  Gain/1 -> [Fx_m]
  Gain1/1 -> [Fz_m]
  My/1 -> Gain2/1
  Gain2/1 -> [My_Iy]
  Product1/1 -> Sum1/1
  [Fz_m] -> Sum1/2
  Sum1/1 -> Integrator1/1, [w_dot]  "w_dot"
  Integrator1/1 -> Integrator4/1, [w]  "w"
  [My_Iy] -> [q_dot], Integrator2/1  "q_dot"
  Integrator2/1 -> Product1/2, [q], Goto5/1, Integrator3/1  "q"
  Integrator3/1 -> Goto4/1  "theta"
  [w] -> MATLAB Function/1(w)
  MATLAB Function/2(alpha) -> [alpha]
  [w_dot] -> MATLAB Function/3(w_dot)
  MATLAB Function/3(alpha_dot) -> [alpha_dot]
  [V] -> Display/1, V/1
  [alpha] -> alpha/1
  [q] -> q/1
  [theta] -> theta/1
  [V_dot] -> V_dot/1
  [alpha_dot] -> alpha_dot/1
  [q_dot] -> q_dot/1
  [theta_dot] -> theta_dot/1
  MATLAB Function/1(V) -> [V]
  MATLAB Function/4(V_dot) -> [V_dot]
  Integrator4/1 -> Goto15/1
  [h] -> h/1
  [w] -> h_dot/1
  [u] -> MATLAB Function/2(u)
  [w_dot] -> w_dot/1
  [u_dot] -> u_dot/1

== system SP_nonlinear_LQR/sefl_built_model_for_verification3/Aero_coefficient ==
  In1 : Inport
  In2 : Inport  Port=2
  In5 : Inport  Port=3
  In7 : Inport  Port=4
  In11 : Inport  Port=5
  In12 : Inport  Port=6
  In13 : Inport  Port=7
  Aerodynamic coefficient : MATLAB Function  TreatAsAtomicUnit=on
  Constant : Constant
  Constant1 : Constant
  Constant2 : Constant
  Mux1 : Mux  Inputs=3
  Mux2 : Mux  Inputs=3
  Out1 : Outport
  Out2 : Outport  Port=2
  wires:
  In5/1 -> Aerodynamic coefficient/3(q)
  In1/1 -> Aerodynamic coefficient/1(vt)
  In2/1 -> Aerodynamic coefficient/2(alpha)
  In7/1 -> Aerodynamic coefficient/4(el)
  Aerodynamic coefficient/3(cmt) -> Mux2/2
  In11/1 -> Aerodynamic coefficient/5(cbar)
  In12/1 -> Aerodynamic coefficient/6(xcgr)
  Aerodynamic coefficient/2(czt) -> Mux1/3
  In13/1 -> Aerodynamic coefficient/7(xcg)
  Aerodynamic coefficient/1(cxt) -> Mux1/1
  Mux1/1 -> Out1/1
  Mux2/1 -> Out2/1
  Constant/1 -> Mux1/2
  Constant1/1 -> Mux2/1
  Constant2/1 -> Mux2/3

== system SP_nonlinear_LQR/sefl_built_model_for_verification3/Flight_dynamics ==
  Fx : Inport
  Fz : Inport  Port=2
  My : Inport  Port=3
  Constant : Constant  Value=op.States(3).x(1)
  Constant1 : Constant  Value=0
  Display : Display
  Gain : Gain  Gain=1/637.1604
  Gain1 : Gain  Gain=1/637.1604
  Gain2 : Gain  Gain=1/55814
  Goto15 : Goto  Commented=on  GotoTag=h
  Goto4 : Goto  Commented=on  GotoTag=theta
  Goto5 : Goto  Commented=on  GotoTag=theta_dot
  Integrator1 : Integrator  InitialCondition=op.States(3).x(2)
  Integrator2 : Integrator
  Integrator3 : Integrator  Commented=on  InitialCondition=op.States(2).x
  Integrator4 : Integrator  Commented=on  InitialCondition=10000
  MATLAB Function : MATLAB Function  TreatAsAtomicUnit=on
  Product1 : Product
  Sum1 : Sum  Inputs=|++
  V : Outport
  alpha : Outport  Port=2
  q : Outport  Port=3
  theta : Outport  Port=4
  h : Outport  Port=5
  V_dot : Outport  Port=6
  alpha_dot : Outport  Port=7
  q_dot : Outport  Port=8
  theta_dot : Outport  Port=9
  h_dot : Outport  Port=10
  w_dot : Outport  Port=11
  u_dot : Outport  Port=12
  wires:
  [u] -> Product1/1
  Constant1/1 -> MATLAB Function/4(u_dot)
  Constant/1 -> [u]
  Fx/1 -> Gain/1
  Fz/1 -> Gain1/1
  Gain/1 -> [Fx_m]
  Gain1/1 -> [Fz_m]
  My/1 -> Gain2/1
  Gain2/1 -> [My_Iy]
  Product1/1 -> Sum1/1
  [Fz_m] -> Sum1/2
  Sum1/1 -> Integrator1/1, [w_dot]  "w_dot"
  Integrator1/1 -> Integrator4/1, [w]  "w"
  [My_Iy] -> [q_dot], Integrator2/1  "q_dot"
  Integrator2/1 -> Product1/2, [q], Goto5/1, Integrator3/1  "q"
  Integrator3/1 -> Goto4/1  "theta"
  [w] -> MATLAB Function/1(w)
  MATLAB Function/2(alpha) -> [alpha]
  [w_dot] -> MATLAB Function/3(w_dot)
  MATLAB Function/3(alpha_dot) -> [alpha_dot]
  [V] -> Display/1, V/1
  [alpha] -> alpha/1
  [q] -> q/1
  [theta] -> theta/1
  [V_dot] -> V_dot/1
  [alpha_dot] -> alpha_dot/1
  [q_dot] -> q_dot/1
  [theta_dot] -> theta_dot/1
  MATLAB Function/1(V) -> [V]
  MATLAB Function/4(V_dot) -> [V_dot]
  Integrator4/1 -> Goto15/1
  [h] -> h/1
  [w] -> h_dot/1
  [u] -> MATLAB Function/2(u)
  [w_dot] -> w_dot/1
  [u_dot] -> u_dot/1

== system SP_nonlinear_LQR/Subsystem/sefl_built_model/Aero_coefficient ==
  In1 : Inport
  In2 : Inport  Port=2
  In5 : Inport  Port=3
  In7 : Inport  Port=4
  In11 : Inport  Port=5
  In12 : Inport  Port=6
  In13 : Inport  Port=7
  Aerodynamic coefficient : MATLAB Function  TreatAsAtomicUnit=on
  Constant : Constant
  Constant1 : Constant
  Constant2 : Constant
  Mux1 : Mux  Inputs=3
  Mux2 : Mux  Inputs=3
  Out1 : Outport
  Out2 : Outport  Port=2
  wires:
  Constant2/1 -> Mux2/3
  Constant1/1 -> Mux2/1
  Constant/1 -> Mux1/2
  Mux2/1 -> Out2/1
  Mux1/1 -> Out1/1
  Aerodynamic coefficient/1(cxt) -> Mux1/1
  In13/1 -> Aerodynamic coefficient/7(xcg)
  Aerodynamic coefficient/2(czt) -> Mux1/3
  In12/1 -> Aerodynamic coefficient/6(xcgr)
  In11/1 -> Aerodynamic coefficient/5(cbar)
  Aerodynamic coefficient/3(cmt) -> Mux2/2
  In7/1 -> Aerodynamic coefficient/4(el)
  In2/1 -> Aerodynamic coefficient/2(alpha)
  In1/1 -> Aerodynamic coefficient/1(vt)
  In5/1 -> Aerodynamic coefficient/3(q)

== system SP_nonlinear_LQR/Subsystem/sefl_built_model/Flight_dynamics ==
  Fx : Inport
  Fz : Inport  Port=2
  My : Inport  Port=3
  w : Inport  Port=4
  q : Inport  Port=5
  Constant : Constant  Value=op.States(3).x(1)
  Constant1 : Constant  Value=0
  Display : Display
  Gain : Gain  Gain=1/637.1604
  Gain1 : Gain  Gain=1/637.1604
  Gain2 : Gain  Gain=1/55814
  MATLAB Function : MATLAB Function  TreatAsAtomicUnit=on
  Product1 : Product
  Sum1 : Sum  Inputs=|++
  V : Outport
  alpha : Outport  Port=2
  theta : Outport  Port=3
  h : Outport  Port=4
  V_dot : Outport  Port=5
  alpha_dot : Outport  Port=6
  q_dot : Outport  Port=7
  theta_dot : Outport  Port=8
  h_dot : Outport  Port=9
  w_dot : Outport  Port=10
  u_dot : Outport  Port=11
  wires:
  [u_dot] -> u_dot/1
  [w_dot] -> w_dot/1
  [u] -> MATLAB Function/2(u)
  [W] -> h_dot/1
  [h] -> h/1
  MATLAB Function/4(V_dot) -> [V_dot]
  MATLAB Function/1(V) -> [V]
  [theta_dot] -> theta_dot/1
  [q_dot] -> q_dot/1
  [alpha_dot] -> alpha_dot/1
  [V_dot] -> V_dot/1
  [theta] -> theta/1
  [alpha] -> alpha/1
  [V] -> V/1, Display/1
  MATLAB Function/3(alpha_dot) -> [alpha_dot]
  [w_dot] -> MATLAB Function/3(w_dot)
  MATLAB Function/2(alpha) -> [alpha]
  [W] -> MATLAB Function/1(w)
  [My_Iy] -> [q_dot]  "q_dot"
  Sum1/1 -> [w_dot]
  [Fz_m] -> Sum1/2
  Product1/1 -> Sum1/1
  Gain2/1 -> [My_Iy]
  My/1 -> Gain2/1
  Gain1/1 -> [Fz_m]
  Gain/1 -> [Fx_m]
  Fz/1 -> Gain1/1
  Fx/1 -> Gain/1
  Constant/1 -> [u]
  Constant1/1 -> MATLAB Function/4(u_dot)
  [u] -> Product1/1
  w/1 -> [W]
  q/1 -> Product1/2
